simulink model "Simulacao_CubeSat_2U"  (R2020a)
settings: Solver=ode45  StartTime=0.0  StopTime=60  MaxStep=1e-4  MinStep=1e-6  RelTol=1e-3
values from neighbouring files (symbols this model uses):
  J = 14e-6    (= 1.4e-05)    [Parametros_Simulacao.m]
  Jb = J + eye(3)*Jc    [Parametros_Simulacao.m]
  Kb = 1/Kv    (= 0.000787940379404)    [Parametros_Simulacao.m]
  Kf = 207.88e-9    (= 2.0788e-07)    [Parametros_Simulacao.m]
  Km = 60/(2*pi*Kv)    (= 0.00752427637463)    [Parametros_Simulacao.m]
  L = 0.05e-3    (= 5e-05)    [Parametros_Simulacao.m]
  R = 0.7    [Parametros_Simulacao.m]
  Te = 0    [Parametros_Simulacao.m]
  Wo = [0 0 (2*vo*pi)/60]'    [Parametros_Simulacao.m]
libraries: simulink x7, sharedutil x1, vrlib x1, aerolibutil x1
settings Model: Creator=gucos  LastModifiedBy=gucos
settings SolverCC: InitialStep=1e-6
settings OptimizationCC: OptimizeBlockIOStorage=off  BufferReuse=off  OptimizeDataStoreBuffers=off  BusAssignmentInplaceUpdate=off
settings DebuggingCC: SFUnexpectedBacktrackingDiag=warning  SFNoUnconditionalDefaultTransitionDiag=warning
settings HardwareCC: ProdBitPerPointer=32  ProdBitPerSizeT=32  ProdBitPerPtrDiffT=32  ProdWordSize=32  ProdHWDeviceType=Intel->x86-32 (Windows32)
settings RTWCC: GenCodeOnly=on  GenerateReport=on  BuildConfiguration=Debug  LaunchReport=on
settings CodeAppCC: ForceParamTrailComments=on  MATLABSourceComments=on  EnableCustomComments=on
settings GRTTargetCC: CombineSignalStateStructs=on  SupportVariableSizeSignals=on  MultiInstanceErrorCode=Warning

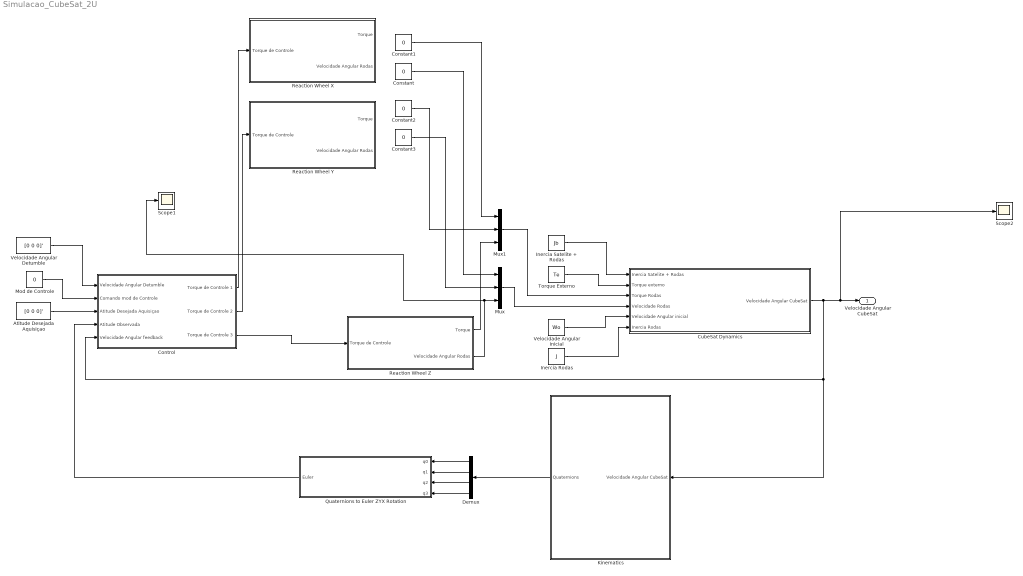
== system Simulacao_CubeSat_2U ==
  Atitude Desejada Aquisiçao : Constant  Value=[0 0 0]'
  Constant{,1..3} (4 alike) : Constant  Value=0
  Control : Subsystem
  CubeSat Dynamics : Subsystem
  Demux : Demux
  Inercia Rodas : Constant  Value=J
  Inercia Satelite + Rodas : Constant  Value=Jb
  Kinematics : Subsystem
  Mod de Controle : Constant  Value=0
  Mux : Mux  Inputs=3
  Mux1 : Mux  Inputs=3
  Quaternions to Euler ZYX Rotation : MATLAB Function  TreatAsAtomicUnit=on
  Reaction Wheel X : Subsystem
  Reaction Wheel Y : Subsystem
  Reaction Wheel Z : Subsystem
  Scope1 : Scope
  Scope2 : Scope
  Torque Externo : Constant  Value=Te
  Velocidade Angular Detumble : Constant  Value=[0 0 0]'
  Velocidade Angular Inicial : Constant  Value=Wo
  Velocidade Angular CubeSat : Outport
  wires:
  Inercia Satelite + Rodas/1 -> CubeSat Dynamics/1(Inercia Satelite + Rodas)
  Torque Externo/1 -> CubeSat Dynamics/2(Torque externo)
  Velocidade Angular Inicial/1 -> CubeSat Dynamics/5(Velocidade Angular inicial)
  Inercia Rodas/1 -> CubeSat Dynamics/6(Inercia Rodas)
  Velocidade Angular Detumble/1 -> Control/1(Velocidade Angular Detumble)
  Atitude Desejada Aquisiçao/1 -> Control/3(Atitude Desejada Aquisiçao)
  CubeSat Dynamics/1(Velocidade Angular CubeSat) -> Scope2/1, Velocidade Angular CubeSat/1, Kinematics/1(Velocidade Angular CubeSat), Control/5(Velocidade Angular feedback)
  Kinematics/1(Quaternions) -> Demux/1
  Demux/4 -> Quaternions to Euler ZYX Rotation/4(q3)
  Demux/3 -> Quaternions to Euler ZYX Rotation/3(q2)
  Demux/1 -> Quaternions to Euler ZYX Rotation/1(q0)
  Demux/2 -> Quaternions to Euler ZYX Rotation/2(q1)
  Control/1(Torque de Controle 1) -> Reaction Wheel X/1(Torque de Controle)
  Reaction Wheel Z/2(Velocidade Angular Rodas) -> Scope1/1, Mux/3
  Reaction Wheel Z/1(Torque) -> Mux1/3
  Mux1/1 -> CubeSat Dynamics/3(Torque Rodas)
  Mux/1 -> CubeSat Dynamics/4(Velocidade Rodas)
  Mod de Controle/1 -> Control/2(Comando mod de Controle)
  Control/2(Torque de Controle 2) -> Reaction Wheel Y/1(Torque de Controle)
  Control/3(Torque de Controle 3) -> Reaction Wheel Z/1(Torque de Controle)
  Quaternions to Euler ZYX Rotation/1(Euler) -> Control/4(Atitude Observada)
  Constant3/1 -> Mux/2
  Constant/1 -> Mux/1
  Constant2/1 -> Mux1/2
  Constant1/1 -> Mux1/1

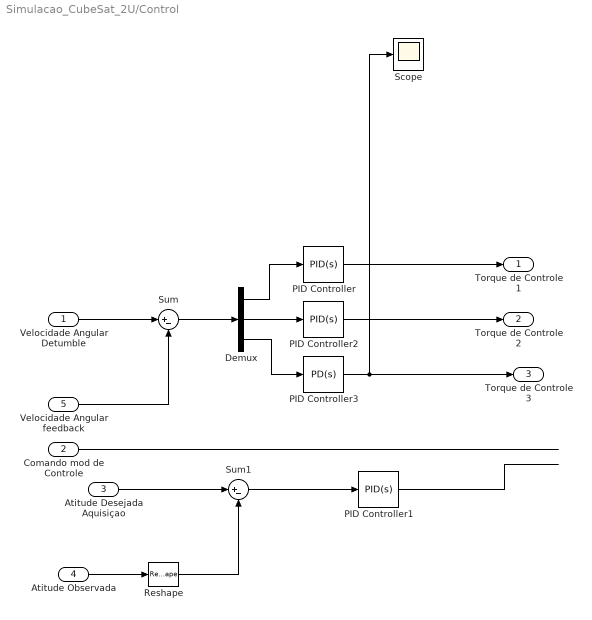
== system Simulacao_CubeSat_2U/Control ==
  Velocidade Angular Detumble : Inport
  Comando mod de Controle : Inport  Port=2
  Atitude Desejada Aquisiçao : Inport  Port=3
  Atitude Observada : Inport  Port=4
  Velocidade Angular feedback : Inport  Port=5
  Demux : Demux  Outputs=3
  PID Controller : simulink/Continuous/PID Controller  Controller=PID  Form=Parallel  TimeDomain=Continuous-time  UseExternalTs=off  SampleTime=-1  IntegratorMethod=Forward Euler  FilterMethod=Forward Euler  ControllerParametersSource=internal  P=-77.8245404530646  I=-0.136815791343329  D=-902.72820032709  UseFilter=on  N=0.0564868262608729  TunerSelectOption=Transfer Function Based (PID Tuner App)  InitialConditionSource=internal  InitialConditionForIntegrator=0  InitialConditionForFilter=0  DifferentiatorICPrevScaledInput=0  ExternalReset=none  TrackingMode=off  Kt=1  LimitOutput=off  UpperSaturationLimit=inf  LowerSaturationLimit=-inf  LinearizeAsGain=on  AntiWindupMode=none  Kb=1  POutMin=[]  POutMax=[]  IOutMin=[]  IOutMax=[]  DOutMin=[]  DOutMax=[]  NOutMin=[]  NOutMax=[]  SumOutMin=[]  SumOutMax=[]  SaturationOutMin=[]  SaturationOutMax=[]  PParamMin=[]  PParamMax=[]  IParamMin=[]  IParamMax=[]  DParamMin=[]  DParamMax=[]  NParamMin=[]  NParamMax=[]  KbParamMin=[]  KbParamMax=[]  KtParamMin=[]  KtParamMax=[]  KbOutMin=[]  KbOutMax=[]  KtOutMin=[]  KtOutMax=[]  IntegratorOutMin=[]  IntegratorOutMax=[]  FilterOutMin=[]  FilterOutMax=[]  SumI1OutMin=[]  SumI1OutMax=[]  SumI2OutMin=[]  SumI2OutMax=[]  SumI3OutMin=[]  SumI3OutMax=[]  SumI4OutMin=[]  SumI4OutMax=[]  SumDOutMin=[]  SumDOutMax=[]  DifferentiatorOutMin=[]  DifferentiatorOutMax=[]  FilterDiffOutCoefMin=[]  FilterDiffOutCoefMax=[]  ReciprocalOutMin=[]  ReciprocalOutMax=[]  SumDenOutMin=[]  SumDenOutMax=[]  SumNumOutMin=[]  SumNumOutMax=[]  DivideOutMin=[]  DivideOutMax=[]  UdiffTsProdOutMin=[]  UdiffTsProdOutMax=[]  NTsProdOutMin=[]  NTsProdOutMax=[]  UintegralTsProdOutMin=[]  UintegralTsProdOutMax=[]  UngainTsProdOutMin=[]  UngainTsProdOutMax=[]  IntegratorContinuousStateAttributes=''  IntegratorStateMustResolveToSignalObject=off  IntegratorRTWStateStorageClass=Auto  FilterContinuousStateAttributes=''  FilterStateMustResolveToSignalObject=off  FilterRTWStateStorageClass=Auto  ParallelPVariant=InternalParameters  IdealPVariant=Disabled  IVariant=InternalParameters  DVariant=InternalParameters  IntegratorVariant=Continuous  SatVariant=Disabled  AWVariant=Passthrough  PCopyVariant=Disabled  TRVariant=Disabled  FdbkBlocksVariant=Forward  IdealPFdbkVariant=Disabled  SatFdbkVariant=Disabled  DerivativeFilterVariant=ContFilter  NVariant=InternalParameters  NCopyVariant=Disabled  FilterICVariant=InternalICsFilter  IntegratorICVariant=InternalICs  ExternalResetVariant=Disabled  TRSumVariant=Passthrough  SumFdbkVariant=Disabled  SumVariant=Sum_PID  TsampFilterVariant=InternalTs  TsampNgainVariant=Passthrough  TsampIntegralVariant=Passthrough
  PID Controller1 : simulink/Continuous/PID Controller  Controller=PID  Form=Parallel  TimeDomain=Continuous-time  UseExternalTs=off  SampleTime=-1  IntegratorMethod=Forward Euler  FilterMethod=Forward Euler  ControllerParametersSource=internal  P=1  I=1  D=0  UseFilter=on  N=100  TunerSelectOption=Transfer Function Based (PID Tuner App)  InitialConditionSource=internal  InitialConditionForIntegrator=0  InitialConditionForFilter=0  DifferentiatorICPrevScaledInput=0  ExternalReset=none  TrackingMode=off  Kt=1  LimitOutput=off  UpperSaturationLimit=inf  LowerSaturationLimit=-inf  LinearizeAsGain=on  AntiWindupMode=none  Kb=1  POutMin=[]  POutMax=[]  IOutMin=[]  IOutMax=[]  DOutMin=[]  DOutMax=[]  NOutMin=[]  NOutMax=[]  SumOutMin=[]  SumOutMax=[]  SaturationOutMin=[]  SaturationOutMax=[]  PParamMin=[]  PParamMax=[]  IParamMin=[]  IParamMax=[]  DParamMin=[]  DParamMax=[]  NParamMin=[]  NParamMax=[]  KbParamMin=[]  KbParamMax=[]  KtParamMin=[]  KtParamMax=[]  KbOutMin=[]  KbOutMax=[]  KtOutMin=[]  KtOutMax=[]  IntegratorOutMin=[]  IntegratorOutMax=[]  FilterOutMin=[]  FilterOutMax=[]  SumI1OutMin=[]  SumI1OutMax=[]  SumI2OutMin=[]  SumI2OutMax=[]  SumI3OutMin=[]  SumI3OutMax=[]  SumI4OutMin=[]  SumI4OutMax=[]  SumDOutMin=[]  SumDOutMax=[]  DifferentiatorOutMin=[]  DifferentiatorOutMax=[]  FilterDiffOutCoefMin=[]  FilterDiffOutCoefMax=[]  ReciprocalOutMin=[]  ReciprocalOutMax=[]  SumDenOutMin=[]  SumDenOutMax=[]  SumNumOutMin=[]  SumNumOutMax=[]  DivideOutMin=[]  DivideOutMax=[]  UdiffTsProdOutMin=[]  UdiffTsProdOutMax=[]  NTsProdOutMin=[]  NTsProdOutMax=[]  UintegralTsProdOutMin=[]  UintegralTsProdOutMax=[]  UngainTsProdOutMin=[]  UngainTsProdOutMax=[]  IntegratorContinuousStateAttributes=''  IntegratorStateMustResolveToSignalObject=off  IntegratorRTWStateStorageClass=Auto  FilterContinuousStateAttributes=''  FilterStateMustResolveToSignalObject=off  FilterRTWStateStorageClass=Auto  ParallelPVariant=InternalParameters  IdealPVariant=Disabled  IVariant=InternalParameters  DVariant=InternalParameters  IntegratorVariant=Continuous  SatVariant=Disabled  AWVariant=Passthrough  PCopyVariant=Disabled  TRVariant=Disabled  FdbkBlocksVariant=Forward  IdealPFdbkVariant=Disabled  SatFdbkVariant=Disabled  DerivativeFilterVariant=ContFilter  NVariant=InternalParameters  NCopyVariant=Disabled  FilterICVariant=InternalICsFilter  IntegratorICVariant=InternalICs  ExternalResetVariant=Disabled  TRSumVariant=Passthrough  SumFdbkVariant=Disabled  SumVariant=Sum_PID  TsampFilterVariant=InternalTs  TsampNgainVariant=Passthrough  TsampIntegralVariant=Passthrough
  PID Controller2 : simulink/Continuous/PID Controller  Controller=PID  Form=Parallel  TimeDomain=Continuous-time  UseExternalTs=off  SampleTime=-1  IntegratorMethod=Forward Euler  FilterMethod=Forward Euler  ControllerParametersSource=internal  P=-10.0233367769767  I=-0.15136600240363  D=-147.47461639554  UseFilter=on  N=295.825597643187  TunerSelectOption=Transfer Function Based (PID Tuner App)  InitialConditionSource=internal  InitialConditionForIntegrator=0  InitialConditionForFilter=0  DifferentiatorICPrevScaledInput=0  ExternalReset=none  TrackingMode=off  Kt=1  LimitOutput=off  UpperSaturationLimit=inf  LowerSaturationLimit=-inf  LinearizeAsGain=on  AntiWindupMode=none  Kb=1  POutMin=[]  POutMax=[]  IOutMin=[]  IOutMax=[]  DOutMin=[]  DOutMax=[]  NOutMin=[]  NOutMax=[]  SumOutMin=[]  SumOutMax=[]  SaturationOutMin=[]  SaturationOutMax=[]  PParamMin=[]  PParamMax=[]  IParamMin=[]  IParamMax=[]  DParamMin=[]  DParamMax=[]  NParamMin=[]  NParamMax=[]  KbParamMin=[]  KbParamMax=[]  KtParamMin=[]  KtParamMax=[]  KbOutMin=[]  KbOutMax=[]  KtOutMin=[]  KtOutMax=[]  IntegratorOutMin=[]  IntegratorOutMax=[]  FilterOutMin=[]  FilterOutMax=[]  SumI1OutMin=[]  SumI1OutMax=[]  SumI2OutMin=[]  SumI2OutMax=[]  SumI3OutMin=[]  SumI3OutMax=[]  SumI4OutMin=[]  SumI4OutMax=[]  SumDOutMin=[]  SumDOutMax=[]  DifferentiatorOutMin=[]  DifferentiatorOutMax=[]  FilterDiffOutCoefMin=[]  FilterDiffOutCoefMax=[]  ReciprocalOutMin=[]  ReciprocalOutMax=[]  SumDenOutMin=[]  SumDenOutMax=[]  SumNumOutMin=[]  SumNumOutMax=[]  DivideOutMin=[]  DivideOutMax=[]  UdiffTsProdOutMin=[]  UdiffTsProdOutMax=[]  NTsProdOutMin=[]  NTsProdOutMax=[]  UintegralTsProdOutMin=[]  UintegralTsProdOutMax=[]  UngainTsProdOutMin=[]  UngainTsProdOutMax=[]  IntegratorContinuousStateAttributes=''  IntegratorStateMustResolveToSignalObject=off  IntegratorRTWStateStorageClass=Auto  FilterContinuousStateAttributes=''  FilterStateMustResolveToSignalObject=off  FilterRTWStateStorageClass=Auto  ParallelPVariant=InternalParameters  IdealPVariant=Disabled  IVariant=InternalParameters  DVariant=InternalParameters  IntegratorVariant=Continuous  SatVariant=Disabled  AWVariant=Passthrough  PCopyVariant=Disabled  TRVariant=Disabled  FdbkBlocksVariant=Forward  IdealPFdbkVariant=Disabled  SatFdbkVariant=Disabled  DerivativeFilterVariant=ContFilter  NVariant=InternalParameters  NCopyVariant=Disabled  FilterICVariant=InternalICsFilter  IntegratorICVariant=InternalICs  ExternalResetVariant=Disabled  TRSumVariant=Passthrough  SumFdbkVariant=Disabled  SumVariant=Sum_PID  TsampFilterVariant=InternalTs  TsampNgainVariant=Passthrough  TsampIntegralVariant=Passthrough
  PID Controller3 : simulink/Continuous/PID Controller  Controller=PD  Form=Parallel  TimeDomain=Continuous-time  UseExternalTs=off  SampleTime=-1  IntegratorMethod=Forward Euler  FilterMethod=Forward Euler  ControllerParametersSource=internal  P=-222578.923246105  I=-169.042119561494  D=-1297.70952411978  UseFilter=on  N=47.294609837714  TunerSelectOption=Transfer Function Based (PID Tuner App)  InitialConditionSource=internal  InitialConditionForIntegrator=0  InitialConditionForFilter=0  DifferentiatorICPrevScaledInput=0  ExternalReset=none  TrackingMode=off  Kt=1  LimitOutput=off  UpperSaturationLimit=inf  LowerSaturationLimit=-inf  LinearizeAsGain=on  AntiWindupMode=none  Kb=1  POutMin=[]  POutMax=[]  IOutMin=[]  IOutMax=[]  DOutMin=[]  DOutMax=[]  NOutMin=[]  NOutMax=[]  SumOutMin=[]  SumOutMax=[]  SaturationOutMin=[]  SaturationOutMax=[]  PParamMin=[]  PParamMax=[]  IParamMin=[]  IParamMax=[]  DParamMin=[]  DParamMax=[]  NParamMin=[]  NParamMax=[]  KbParamMin=[]  KbParamMax=[]  KtParamMin=[]  KtParamMax=[]  KbOutMin=[]  KbOutMax=[]  KtOutMin=[]  KtOutMax=[]  IntegratorOutMin=[]  IntegratorOutMax=[]  FilterOutMin=[]  FilterOutMax=[]  SumI1OutMin=[]  SumI1OutMax=[]  SumI2OutMin=[]  SumI2OutMax=[]  SumI3OutMin=[]  SumI3OutMax=[]  SumI4OutMin=[]  SumI4OutMax=[]  SumDOutMin=[]  SumDOutMax=[]  DifferentiatorOutMin=[]  DifferentiatorOutMax=[]  FilterDiffOutCoefMin=[]  FilterDiffOutCoefMax=[]  ReciprocalOutMin=[]  ReciprocalOutMax=[]  SumDenOutMin=[]  SumDenOutMax=[]  SumNumOutMin=[]  SumNumOutMax=[]  DivideOutMin=[]  DivideOutMax=[]  UdiffTsProdOutMin=[]  UdiffTsProdOutMax=[]  NTsProdOutMin=[]  NTsProdOutMax=[]  UintegralTsProdOutMin=[]  UintegralTsProdOutMax=[]  UngainTsProdOutMin=[]  UngainTsProdOutMax=[]  IntegratorContinuousStateAttributes=''  IntegratorStateMustResolveToSignalObject=off  IntegratorRTWStateStorageClass=Auto  FilterContinuousStateAttributes=''  FilterStateMustResolveToSignalObject=off  FilterRTWStateStorageClass=Auto  ParallelPVariant=InternalParameters  IdealPVariant=Disabled  IVariant=Disabled  DVariant=InternalParameters  IntegratorVariant=Disabled  SatVariant=Disabled  AWVariant=Disabled  PCopyVariant=Disabled  TRVariant=Disabled  FdbkBlocksVariant=Forward  IdealPFdbkVariant=Disabled  SatFdbkVariant=Disabled  DerivativeFilterVariant=ContFilter  NVariant=InternalParameters  NCopyVariant=Disabled  FilterICVariant=InternalICsFilter  IntegratorICVariant=Disabled  ExternalResetVariant=Disabled  TRSumVariant=Passthrough  SumFdbkVariant=Disabled  SumVariant=Sum_PD  TsampFilterVariant=InternalTs  TsampNgainVariant=Passthrough  TsampIntegralVariant=Disabled_SignalSpec
  Reshape : Reshape  OutputDimensionality=Column vector (2-D)
  Scope : Scope
  Sum : Sum  Inputs=|+-
  Sum1 : Sum  Inputs=|+-
  Torque de Controle 1 : Outport
  Torque de Controle 2 : Outport  Port=2
  Torque de Controle 3 : Outport  Port=3
  wires:
  Velocidade Angular feedback/1 -> Sum/2
  Velocidade Angular Detumble/1 -> Sum/1
  Sum1/1 -> PID Controller1/1
  Atitude Desejada Aquisiçao/1 -> Sum1/1
  Atitude Observada/1 -> Reshape/1
  Reshape/1 -> Sum1/2
  PID Controller/1 -> Torque de Controle 1/1
  Sum/1 -> Demux/1
  Demux/1 -> PID Controller/1
  Demux/2 -> PID Controller2/1
  Demux/3 -> PID Controller3/1
  PID Controller2/1 -> Torque de Controle 2/1
  PID Controller3/1 -> Torque de Controle 3/1, Scope/1
  PID Controller1/1 -> ?
  Comando mod de Controle/1 -> ?

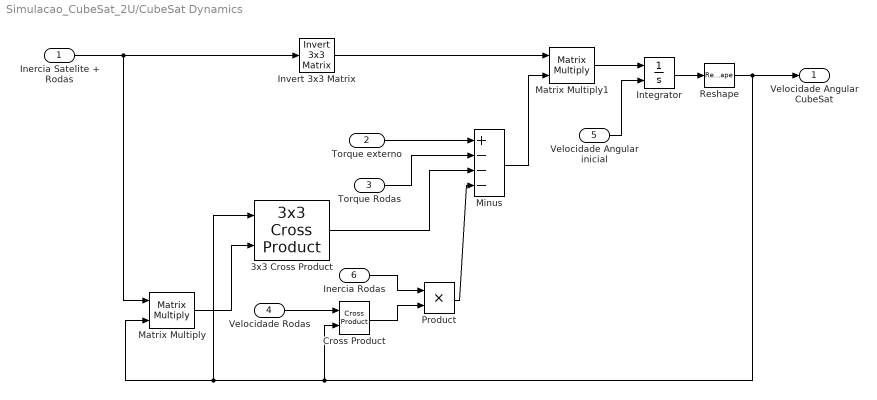
== system Simulacao_CubeSat_2U/CubeSat Dynamics ==
  Inercia Satelite + Rodas : Inport
  Torque externo : Inport  Port=2
  Torque Rodas : Inport  Port=3
  Velocidade Rodas : Inport  Port=4
  Velocidade Angular inicial : Inport  Port=5
  Inercia Rodas : Inport  Port=6
  3x3 Cross Product : sharedutil/3x3 Cross Product  aMode=aMode
      settings: SourceProductBaseCode=AE,PW,MT,VE,VP
  Cross Product : vrlib/Utilities/Cross Product
  Integrator : Integrator  InitialConditionSource=external
  Invert 3x3 Matrix : aerolibutil/Invert  3x3 Matrix
  Matrix Multiply : Product  Multiplication=Matrix(*)
  Matrix Multiply1 : Product  Multiplication=Matrix(*)
  Minus : Sum  Inputs=+---
  Product : Product
  Reshape : Reshape  OutputDimensionality=Column vector (2-D)  OutputDimensions=[,1]
  Velocidade Angular CubeSat : Outport
  wires:
  Velocidade Rodas/1 -> Cross Product/1
  Invert 3x3 Matrix/1 -> Matrix Multiply1/1
  3x3 Cross Product/1 -> Minus/3
  Inercia Satelite + Rodas/1 -> Matrix Multiply/1, Invert 3x3 Matrix/1
  Velocidade Angular inicial/1 -> Integrator/2
  Matrix Multiply/1 -> 3x3 Cross Product/2
  Torque externo/1 -> Minus/1
  Minus/1 -> Matrix Multiply1/2
  Matrix Multiply1/1 -> Integrator/1
  Torque Rodas/1 -> Minus/2
  Product/1 -> Minus/4
  Cross Product/1 -> Product/2
  Inercia Rodas/1 -> Product/1
  Reshape/1 -> Velocidade Angular CubeSat/1, Cross Product/2, 3x3 Cross Product/1, Matrix Multiply/2
  Integrator/1 -> Reshape/1

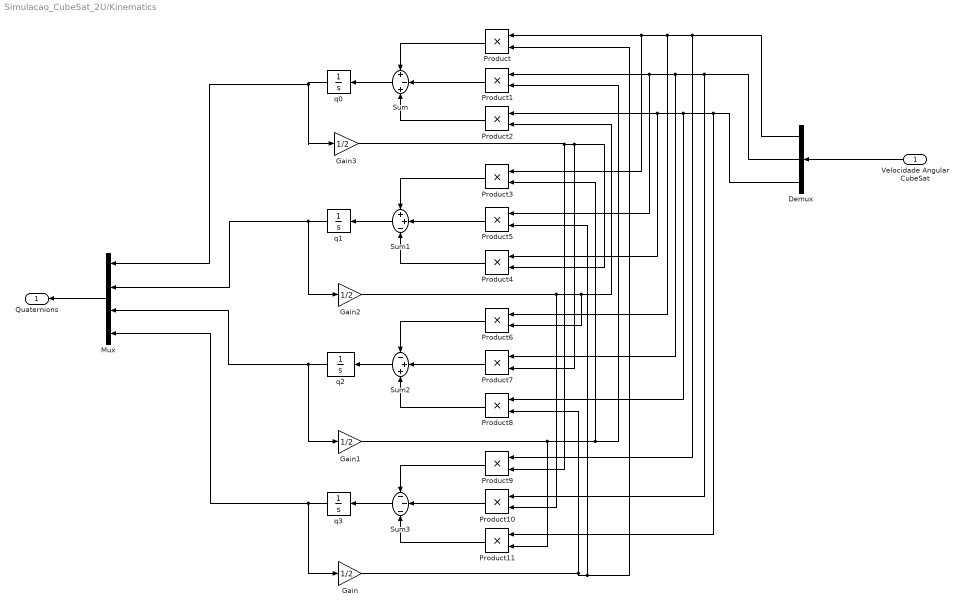
== system Simulacao_CubeSat_2U/Kinematics ==
  Velocidade Angular CubeSat : Inport
  Demux : Demux  Outputs=3
  Gain{,1..3} (4 alike) : Gain  Gain=1/2
  Mux : Mux
  Product{,1..11} (12 alike) : Product
  Sum : Sum  Inputs=+-+
  Sum1 : Sum  Inputs=++-
  Sum2 : Sum  Inputs=-++
  Sum3 : Sum  Inputs=---
  q0 : Integrator  InitialCondition=-1
  q1 : Integrator
  q2 : Integrator
  q3 : Integrator
  Quaternions : Outport
  wires:
  Demux/2 -> Product10/1, Product7/1, Product5/1, Product1/1
  Demux/3 -> Product11/1, Product8/1, Product4/1, Product2/1
  q0/1 -> Gain3/1, Mux/1
  q2/1 -> Mux/3, Gain1/1
  Product9/1 -> Sum3/1
  Product7/1 -> Sum2/2
  q1/1 -> Gain2/1, Mux/2
  Velocidade Angular CubeSat/1 -> Demux/1
  Product4/1 -> Sum1/3
  Mux/1 -> Quaternions/1
  Sum2/1 -> q2/1
  q3/1 -> Mux/4, Gain/1
  Sum1/1 -> q1/1
  Product5/1 -> Sum1/2
  Product/1 -> Sum/1
  Product3/1 -> Sum1/1
  Product2/1 -> Sum/3
  Sum3/1 -> q3/1
  Demux/1 -> Product9/1, Product6/1, Product3/1, Product/1
  Product1/1 -> Sum/2
  Product8/1 -> Sum2/3
  Product10/1 -> Sum3/2
  Product11/1 -> Sum3/3
  Sum/1 -> q0/1
  Product6/1 -> Sum2/1
  Gain3/1 -> Product9/2, Product7/2, Product4/2
  Gain2/1 -> Product10/2, Product6/2, Product2/2
  Gain1/1 -> Product11/2, Product3/2, Product1/2
  Gain/1 -> Product5/2, Product/2, Product8/2

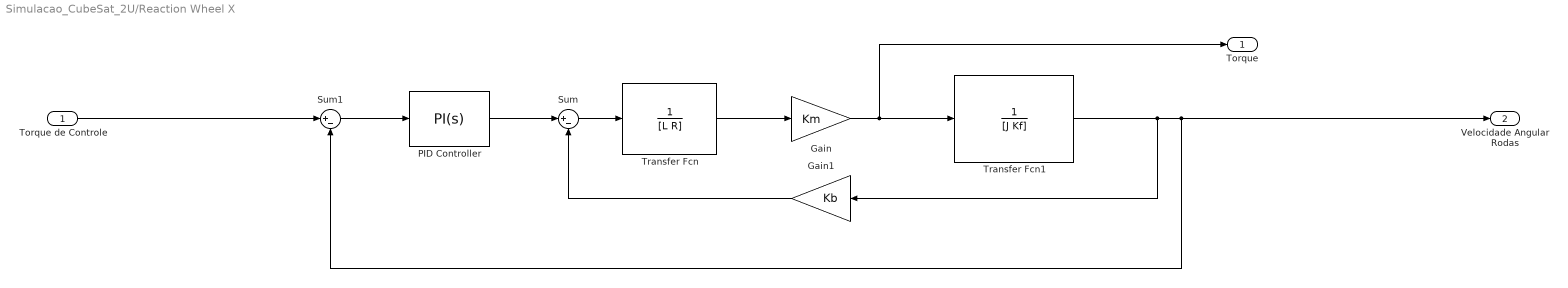
== system Simulacao_CubeSat_2U/Reaction Wheel X ==
  Torque de Controle : Inport
  Gain : Gain  Gain=Km
  Gain1 : Gain  Gain=Kb
  PID Controller : simulink/Continuous/PID Controller  Controller=PI  Form=Parallel  TimeDomain=Continuous-time  UseExternalTs=off  SampleTime=-1  IntegratorMethod=Forward Euler  FilterMethod=Forward Euler  ControllerParametersSource=internal  P=-0.00108347393652397  I=-9.48136485367531e-06  D=0  UseFilter=on  N=100  TunerSelectOption=Transfer Function Based (PID Tuner App)  InitialConditionSource=internal  InitialConditionForIntegrator=0  InitialConditionForFilter=0  DifferentiatorICPrevScaledInput=0  ExternalReset=none  TrackingMode=off  Kt=1  LimitOutput=off  UpperSaturationLimit=inf  LowerSaturationLimit=-inf  LinearizeAsGain=on  AntiWindupMode=none  Kb=1  POutMin=[]  POutMax=[]  IOutMin=[]  IOutMax=[]  DOutMin=[]  DOutMax=[]  NOutMin=[]  NOutMax=[]  SumOutMin=[]  SumOutMax=[]  SaturationOutMin=[]  SaturationOutMax=[]  PParamMin=[]  PParamMax=[]  IParamMin=[]  IParamMax=[]  DParamMin=[]  DParamMax=[]  NParamMin=[]  NParamMax=[]  KbParamMin=[]  KbParamMax=[]  KtParamMin=[]  KtParamMax=[]  KbOutMin=[]  KbOutMax=[]  KtOutMin=[]  KtOutMax=[]  IntegratorOutMin=[]  IntegratorOutMax=[]  FilterOutMin=[]  FilterOutMax=[]  SumI1OutMin=[]  SumI1OutMax=[]  SumI2OutMin=[]  SumI2OutMax=[]  SumI3OutMin=[]  SumI3OutMax=[]  SumI4OutMin=[]  SumI4OutMax=[]  SumDOutMin=[]  SumDOutMax=[]  DifferentiatorOutMin=[]  DifferentiatorOutMax=[]  FilterDiffOutCoefMin=[]  FilterDiffOutCoefMax=[]  ReciprocalOutMin=[]  ReciprocalOutMax=[]  SumDenOutMin=[]  SumDenOutMax=[]  SumNumOutMin=[]  SumNumOutMax=[]  DivideOutMin=[]  DivideOutMax=[]  UdiffTsProdOutMin=[]  UdiffTsProdOutMax=[]  NTsProdOutMin=[]  NTsProdOutMax=[]  UintegralTsProdOutMin=[]  UintegralTsProdOutMax=[]  UngainTsProdOutMin=[]  UngainTsProdOutMax=[]  IntegratorContinuousStateAttributes=''  IntegratorStateMustResolveToSignalObject=off  IntegratorRTWStateStorageClass=Auto  FilterContinuousStateAttributes=''  FilterStateMustResolveToSignalObject=off  FilterRTWStateStorageClass=Auto  ParallelPVariant=InternalParameters  IdealPVariant=Disabled  IVariant=InternalParameters  DVariant=Disabled  IntegratorVariant=Continuous  SatVariant=Disabled  AWVariant=Passthrough  PCopyVariant=Disabled  TRVariant=Disabled  FdbkBlocksVariant=Forward  IdealPFdbkVariant=Disabled  SatFdbkVariant=Disabled  DerivativeFilterVariant=Disabled  NVariant=Disabled  NCopyVariant=Disabled_SignalSpec  FilterICVariant=Disabled  IntegratorICVariant=InternalICs  ExternalResetVariant=Disabled  TRSumVariant=Passthrough  SumFdbkVariant=Disabled  SumVariant=Sum_PI  TsampFilterVariant=InternalTs  TsampNgainVariant=Passthrough  TsampIntegralVariant=Passthrough
  Sum : Sum  Inputs=|+-
  Sum1 : Sum  Inputs=|+-
  Transfer Fcn : TransferFcn  Denominator=[L R]
  Transfer Fcn1 : TransferFcn  Denominator=[J Kf]
  Torque : Outport
  Velocidade Angular Rodas : Outport  Port=2
  wires:
  Gain/1 -> Torque/1, Transfer Fcn1/1
  Transfer Fcn/1 -> Gain/1
  PID Controller/1 -> Sum/1
  Gain1/1 -> Sum/2
  Sum/1 -> Transfer Fcn/1
  Sum1/1 -> PID Controller/1
  Torque de Controle/1 -> Sum1/1
  Transfer Fcn1/1 -> Velocidade Angular Rodas/1, Sum1/2, Gain1/1

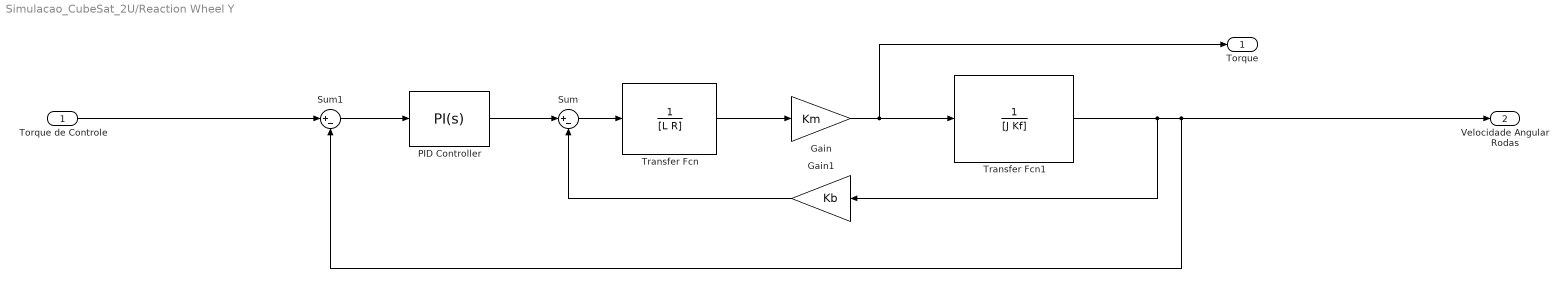
== system Simulacao_CubeSat_2U/Reaction Wheel Y ==
  Torque de Controle : Inport
  Gain : Gain  Gain=Km
  Gain1 : Gain  Gain=Kb
  PID Controller : simulink/Continuous/PID Controller  Controller=PI  Form=Parallel  TimeDomain=Continuous-time  UseExternalTs=off  SampleTime=-1  IntegratorMethod=Forward Euler  FilterMethod=Forward Euler  ControllerParametersSource=internal  P=0.000981777984787663  I=8.59143442706334e-06  D=0  UseFilter=on  N=100  TunerSelectOption=Transfer Function Based (PID Tuner App)  InitialConditionSource=internal  InitialConditionForIntegrator=0  InitialConditionForFilter=0  DifferentiatorICPrevScaledInput=0  ExternalReset=none  TrackingMode=off  Kt=1  LimitOutput=off  UpperSaturationLimit=inf  LowerSaturationLimit=-inf  LinearizeAsGain=on  AntiWindupMode=none  Kb=1  POutMin=[]  POutMax=[]  IOutMin=[]  IOutMax=[]  DOutMin=[]  DOutMax=[]  NOutMin=[]  NOutMax=[]  SumOutMin=[]  SumOutMax=[]  SaturationOutMin=[]  SaturationOutMax=[]  PParamMin=[]  PParamMax=[]  IParamMin=[]  IParamMax=[]  DParamMin=[]  DParamMax=[]  NParamMin=[]  NParamMax=[]  KbParamMin=[]  KbParamMax=[]  KtParamMin=[]  KtParamMax=[]  KbOutMin=[]  KbOutMax=[]  KtOutMin=[]  KtOutMax=[]  IntegratorOutMin=[]  IntegratorOutMax=[]  FilterOutMin=[]  FilterOutMax=[]  SumI1OutMin=[]  SumI1OutMax=[]  SumI2OutMin=[]  SumI2OutMax=[]  SumI3OutMin=[]  SumI3OutMax=[]  SumI4OutMin=[]  SumI4OutMax=[]  SumDOutMin=[]  SumDOutMax=[]  DifferentiatorOutMin=[]  DifferentiatorOutMax=[]  FilterDiffOutCoefMin=[]  FilterDiffOutCoefMax=[]  ReciprocalOutMin=[]  ReciprocalOutMax=[]  SumDenOutMin=[]  SumDenOutMax=[]  SumNumOutMin=[]  SumNumOutMax=[]  DivideOutMin=[]  DivideOutMax=[]  UdiffTsProdOutMin=[]  UdiffTsProdOutMax=[]  NTsProdOutMin=[]  NTsProdOutMax=[]  UintegralTsProdOutMin=[]  UintegralTsProdOutMax=[]  UngainTsProdOutMin=[]  UngainTsProdOutMax=[]  IntegratorContinuousStateAttributes=''  IntegratorStateMustResolveToSignalObject=off  IntegratorRTWStateStorageClass=Auto  FilterContinuousStateAttributes=''  FilterStateMustResolveToSignalObject=off  FilterRTWStateStorageClass=Auto  ParallelPVariant=InternalParameters  IdealPVariant=Disabled  IVariant=InternalParameters  DVariant=Disabled  IntegratorVariant=Continuous  SatVariant=Disabled  AWVariant=Passthrough  PCopyVariant=Disabled  TRVariant=Disabled  FdbkBlocksVariant=Forward  IdealPFdbkVariant=Disabled  SatFdbkVariant=Disabled  DerivativeFilterVariant=Disabled  NVariant=Disabled  NCopyVariant=Disabled_SignalSpec  FilterICVariant=Disabled  IntegratorICVariant=InternalICs  ExternalResetVariant=Disabled  TRSumVariant=Passthrough  SumFdbkVariant=Disabled  SumVariant=Sum_PI  TsampFilterVariant=InternalTs  TsampNgainVariant=Passthrough  TsampIntegralVariant=Passthrough
  Sum : Sum  Inputs=|+-
  Sum1 : Sum  Inputs=|+-
  Transfer Fcn : TransferFcn  Denominator=[L R]
  Transfer Fcn1 : TransferFcn  Denominator=[J Kf]
  Torque : Outport
  Velocidade Angular Rodas : Outport  Port=2
  wires:
  Gain/1 -> Torque/1, Transfer Fcn1/1
  Transfer Fcn/1 -> Gain/1
  PID Controller/1 -> Sum/1
  Gain1/1 -> Sum/2
  Sum/1 -> Transfer Fcn/1
  Sum1/1 -> PID Controller/1
  Torque de Controle/1 -> Sum1/1
  Transfer Fcn1/1 -> Velocidade Angular Rodas/1, Sum1/2, Gain1/1

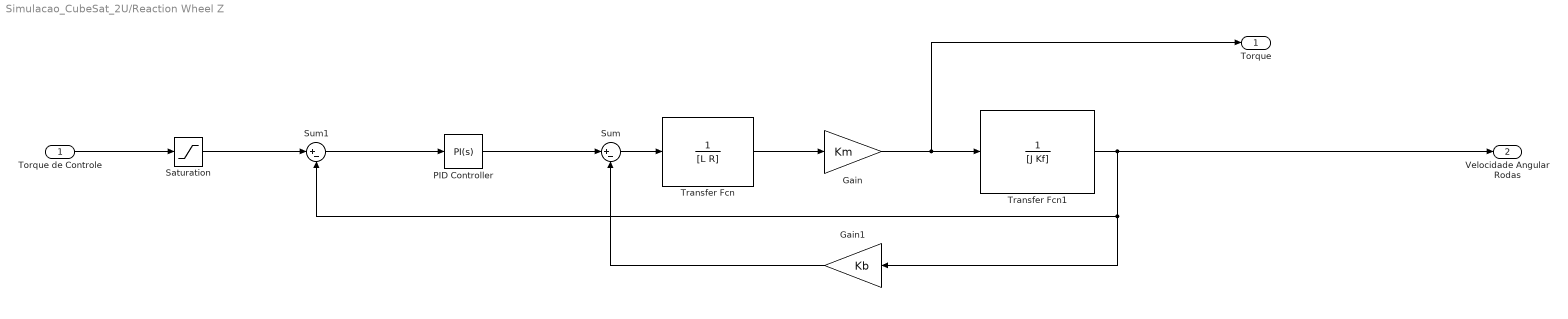
== system Simulacao_CubeSat_2U/Reaction Wheel Z ==
  Torque de Controle : Inport
  Gain : Gain  Gain=Km
  Gain1 : Gain  Gain=Kb
  PID Controller : simulink/Continuous/PID Controller  Controller=PI  Form=Parallel  TimeDomain=Continuous-time  UseExternalTs=off  SampleTime=-1  IntegratorMethod=Forward Euler  FilterMethod=Forward Euler  ControllerParametersSource=internal  P=4.38758194806958e-07  I=1.99671945141145e-06  D=0  UseFilter=on  N=100  TunerSelectOption=Transfer Function Based (PID Tuner App)  InitialConditionSource=internal  InitialConditionForIntegrator=0  InitialConditionForFilter=0  DifferentiatorICPrevScaledInput=0  ExternalReset=none  TrackingMode=off  Kt=1  LimitOutput=off  UpperSaturationLimit=inf  LowerSaturationLimit=-inf  LinearizeAsGain=on  AntiWindupMode=none  Kb=1  POutMin=[]  POutMax=[]  IOutMin=[]  IOutMax=[]  DOutMin=[]  DOutMax=[]  NOutMin=[]  NOutMax=[]  SumOutMin=[]  SumOutMax=[]  SaturationOutMin=[]  SaturationOutMax=[]  PParamMin=[]  PParamMax=[]  IParamMin=[]  IParamMax=[]  DParamMin=[]  DParamMax=[]  NParamMin=[]  NParamMax=[]  KbParamMin=[]  KbParamMax=[]  KtParamMin=[]  KtParamMax=[]  KbOutMin=[]  KbOutMax=[]  KtOutMin=[]  KtOutMax=[]  IntegratorOutMin=[]  IntegratorOutMax=[]  FilterOutMin=[]  FilterOutMax=[]  SumI1OutMin=[]  SumI1OutMax=[]  SumI2OutMin=[]  SumI2OutMax=[]  SumI3OutMin=[]  SumI3OutMax=[]  SumI4OutMin=[]  SumI4OutMax=[]  SumDOutMin=[]  SumDOutMax=[]  DifferentiatorOutMin=[]  DifferentiatorOutMax=[]  FilterDiffOutCoefMin=[]  FilterDiffOutCoefMax=[]  ReciprocalOutMin=[]  ReciprocalOutMax=[]  SumDenOutMin=[]  SumDenOutMax=[]  SumNumOutMin=[]  SumNumOutMax=[]  DivideOutMin=[]  DivideOutMax=[]  UdiffTsProdOutMin=[]  UdiffTsProdOutMax=[]  NTsProdOutMin=[]  NTsProdOutMax=[]  UintegralTsProdOutMin=[]  UintegralTsProdOutMax=[]  UngainTsProdOutMin=[]  UngainTsProdOutMax=[]  IntegratorContinuousStateAttributes=''  IntegratorStateMustResolveToSignalObject=off  IntegratorRTWStateStorageClass=Auto  FilterContinuousStateAttributes=''  FilterStateMustResolveToSignalObject=off  FilterRTWStateStorageClass=Auto  ParallelPVariant=InternalParameters  IdealPVariant=Disabled  IVariant=InternalParameters  DVariant=Disabled  IntegratorVariant=Continuous  SatVariant=Disabled  AWVariant=Passthrough  PCopyVariant=Disabled  TRVariant=Disabled  FdbkBlocksVariant=Forward  IdealPFdbkVariant=Disabled  SatFdbkVariant=Disabled  DerivativeFilterVariant=Disabled  NVariant=Disabled  NCopyVariant=Disabled_SignalSpec  FilterICVariant=Disabled  IntegratorICVariant=InternalICs  ExternalResetVariant=Disabled  TRSumVariant=Passthrough  SumFdbkVariant=Disabled  SumVariant=Sum_PI  TsampFilterVariant=InternalTs  TsampNgainVariant=Passthrough  TsampIntegralVariant=Passthrough
  Saturation : Saturate  UpperLimit=628.3  LowerLimit=-628.3
  Sum : Sum  Inputs=|+-
  Sum1 : Sum  Inputs=|+-
  Transfer Fcn : TransferFcn  Denominator=[L R]
  Transfer Fcn1 : TransferFcn  Denominator=[J Kf]
  Torque : Outport
  Velocidade Angular Rodas : Outport  Port=2
  wires:
  Gain/1 -> Torque/1, Transfer Fcn1/1
  Transfer Fcn/1 -> Gain/1
  Gain1/1 -> Sum/2
  Sum/1 -> Transfer Fcn/1
  Transfer Fcn1/1 -> Sum1/2, Gain1/1, Velocidade Angular Rodas/1
  PID Controller/1 -> Sum/1
  Sum1/1 -> PID Controller/1
  Torque de Controle/1 -> Saturation/1
  Saturation/1 -> Sum1/1

== matlab function Simulacao_CubeSat_2U/Quaternions to Euler ZYX Rotation ==
  data: q0 input; Euler output; q1 input; q2 input; q3 input

function Euler = ZYX(q0, q1, q2, q3)


C11 = (q0^2)+(q1^2)-(q2^2)-(q3^2);
C12 = (2*(q1*q2+q0*q3));
C13 = (2*(q1*q3-q0*q2));
%C21 = 2*(q1*q2-q0*q3)
%C22 = (q0^2)-(q1^2)+(q2^2)-(q3^2)
C23 = (2*(q2*q3+q0*q1));
%C31 = 2*(q1*q3+q0*q2)
%C32 = 2*(q2*q3-q0*q1)
C33 = ((q0^2)-(q1^2)-(q2^2)+(q3^2));

%C = [C11 C12 C13; C21 C22 C23; C31 C32 C33]

%DCM = [ctheta*calpha ctheta*salpha -stheta; sphi*stheta*calpha-cphi*salpha
%sphi*stheta*salpha+cphi*calpha sphi*ctheta; cphi*stheta*calpha+sphi*salpha
%cphi*stheta*salpha-sphi*calpha cphi*calpha]

theta = asind(-C13);


if C12 >= 0 && C11 >= 0
    
    if C23 >= 0 && C33 >= 0

        alpha = atand(C12/C11);
        phi = atand(C23/C33);

    elseif C23 >= 0 && C33 <= 0 

        alpha = atand(C12/C11);
        phi = atand(C23/C33) + 180;
        
    elseif C23 <= 0 && C33 <= 0

         alpha = atand(C12/C11);
         phi = atand(C23/C33) - 180;

    elseif C23 <= 0 && C33 >= 0

        alpha = atand(C12/C11);
        phi = atand(C23/C33);
        
         
    else
        
        alpha = 0;
        phi = 0;


    end

    
elseif C12 >= 0 && C11 <= 0 
    
    if C23 >= 0 && C33 >= 0

        alpha = atand(C12/C11) + 180;
        phi = atand(C23/C33);

    elseif C23 >= 0 && C33 <= 0 

        if q1 == 0 && q3 == 0
            alpha = atand(C12/C11);
            phi = atand(C23/C33);
        else
            alpha = atand(C12/C11) + 180;
            phi = atand(C23/C33) + 180;
        end
        
    elseif C23 <= 0 && C33 <= 0

         alpha = atand(C12/C11) + 180;
         phi = atand(C23/C33) - 180;

    elseif C23 <= 0 && C33 >= 0

        alpha = atand(C12/C11) + 180;
        phi = atand(C23/C33);
        
         
    else
        
        alpha = 0;
        phi = 0;


    end
    
    
elseif C12 <= 0 && C11 <= 0
    
    if C23 >= 0 && C33 >= 0

        alpha = atand(C12/C11) - 180;
        phi = atand(C23/C33);

    elseif C23 >= 0 && C33 <= 0 

        alpha = atand(C12/C11) - 180;
        phi = atand(C23/C33) + 180;
        
    elseif C23 <= 0 && C33 <= 0

         alpha = atand(C12/C11) - 180;
         phi = atand(C23/C33) - 180;

    elseif C23 <= 0 && C33 >= 0

        alpha = atand(C12/C11) - 180;
        phi = atand(C23/C33);
        
         
    else
        
        alpha = 0;
        phi = 0;


    end
     
     
elseif C12 <= 0 && C11 >= 0
    
    if C23 >= 0 && C33 >= 0

        alpha = atand(C12/C11);
        phi = atand(C23/C33);

    elseif C23 >= 0 && C33 <= 0 

        alpha = atand(C12/C11);
        phi = atand(C23/C33) + 180;
        
    elseif C23 <= 0 && C33 <= 0

         alpha = atand(C12/C11);
         phi = atand(C23/C33) - 180;

    elseif C23 <= 0 && C33 >= 0

        alpha = atand(C12/C11);
        phi = atand(C23/C33);
        
    else
        
        alpha = 0;
        phi = 0;

    end
    
else
    
    alpha = 0;
    phi = 0;
    
end

Euler = [alpha theta phi];
end
